simulink model "AC1P2_model"  (R2025b)
settings: Solver=VariableStepAuto  StartTime=0.0  StopTime=10.0  RelTol=1e-3
values from neighbouring files (symbols this model uses):
  c1 = 2    [AC1P2_script.m]
  k1 = 4    [AC1P2_script.m]
  k2 = 20    [AC1P2_script.m]
  m1 = 2    [AC1P2_script.m]
  m2 = 5    [AC1P2_script.m]
libraries: simulink x1
settings Model: Creator=micha  LastModifiedBy=micha

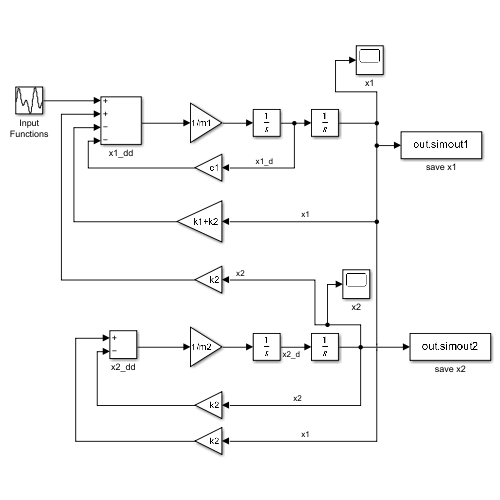
[thumbnail: Simulink's stored preview of the top-level diagram]
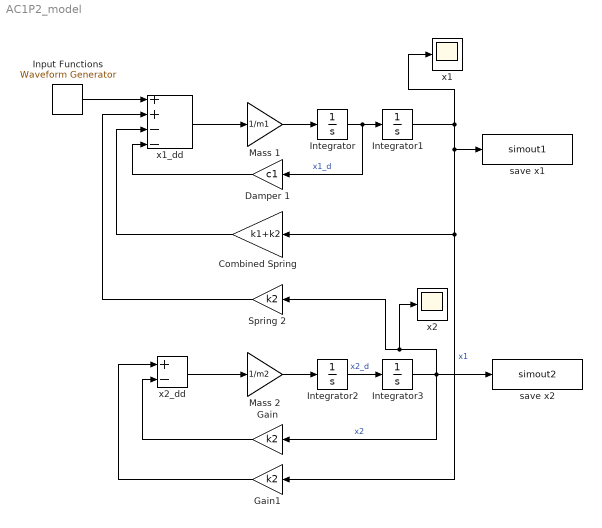
== system AC1P2_model ==
  Combined Spring : Gain  Gain=k1+k2
  Damper 1 : Gain  Gain=c1
  Gain : Gain  Gain=k2
  Gain1 : Gain  Gain=k2
  Input Functions : simulink/Sources/Waveform Generator  OutMin=[]  OutMax=[]  OutDataTypeStr=double  SelectedSignal=4  Signals=step(1, 0, 1)#sin('Amplitude', 1, 'Frequency', 1.41421356, 'Phase', 0)#sin(1, 2, 0)#sin(1, 5, 0)  BlockNames=MultiportSwitch_95980429a43848d#MultiportSwitch_445d85ad0d254f2#MultiportSwitch_0e1d35064a3a4b7#MultiportSwitch_2ec384411d39472  SampleTime=0.1
  Integrator{,1..3} (4 alike) : Integrator
  Mass 1 : Gain  Gain=1/m1
  Mass 2 : Gain  Gain=1/m2
  Spring 2 : Gain  Gain=k2
  save x1 : ToWorkspace  VariableName=simout1  SaveFormat=Timeseries  SampleTime=-1
  save x2 : ToWorkspace  VariableName=simout2  SaveFormat=Timeseries  SampleTime=-1
  x1 : Scope
      settings: ActiveDisplayYMinimum=-1  ActiveDisplayYMaximum=1
  x1_dd : Sum  Inputs=++--
  x2 : Scope
  x2_dd : Sum  Inputs=+-
  wires:
  Input Functions/1 -> x1_dd/1
  x1_dd/1 -> Mass 1/1
  Damper 1/1 -> x1_dd/4
  Spring 2/1 -> x1_dd/2
  Combined Spring/1 -> x1_dd/3
  Mass 1/1 -> Integrator/1
  Integrator/1 -> Damper 1/1, Integrator1/1  "x1_d"
  Integrator1/1 -> save x1/1, Combined Spring/1, Gain1/1, x1/1  "x1"
  Integrator3/1 -> save x2/1, Spring 2/1, x2/1, Gain/1  "x2"
  x2_dd/1 -> Mass 2/1
  Gain/1 -> x2_dd/2
  Mass 2/1 -> Integrator2/1
  Gain1/1 -> x2_dd/1
  Integrator2/1 -> Integrator3/1  "x2_d"
